simulink model "week2_problem4_2005052"  (R2021a)
settings: Solver=VariableStepAuto  StartTime=0.0  StopTime=10.0  RelTol=1e-3
model workspace (MAT data in the model file):
  B = 50
  J = Simulink.Parameter
  J.Value = 3.2284e-06
  J.DataType = 'auto'
  J.Dimensions = [1 1]
  Kd = 484.0516
  Ke = Simulink.Parameter
  Ke.Value = 0.0274
  Ke.DataType = 'auto'
  Ke.Dimensions = [1 1]
  Ki = 83.0917
  Kp = 495.0505
  Kt = Simulink.Parameter
  Kt.Value = 0.0274
  Kt.DataType = 'auto'
  Kt.Dimensions = [1 1]
  L = Simulink.Parameter
  L.Value = 2.75e-06
  L.DataType = 'auto'
  L.Dimensions = [1 1]
  M = 1000
  R = Simulink.Parameter
  R.Value = 4
  R.DataType = 'auto'
  R.Dimensions = [1 1]
  Ts = Simulink.Parameter
  Ts.Value = 0.01
  Ts.DataType = 'auto'
  Ts.Dimensions = [1 1]
  b = Simulink.Parameter
  b.Value = 3.5077e-06
  b.DataType = 'auto'
  b.Dimensions = [1 1]
  kd = Simulink.Parameter
  kd.Value = 50
  kd.DataType = 'auto'
  kd.Dimensions = [1 1]
  ki = Simulink.Parameter
  ki.Value = 22000
  ki.DataType = 'auto'
  ki.Dimensions = [1 1]
  kp = Simulink.Parameter
  kp.Value = 22000
  kp.DataType = 'auto'
  kp.Dimensions = [1 1]
settings Model: Creator=admin  LastModifiedBy=admin
settings SolverCC: AlgebraicLoopSolver=TrustRegion
settings DebuggingCC: SFMachineParentedDataDiag=warning

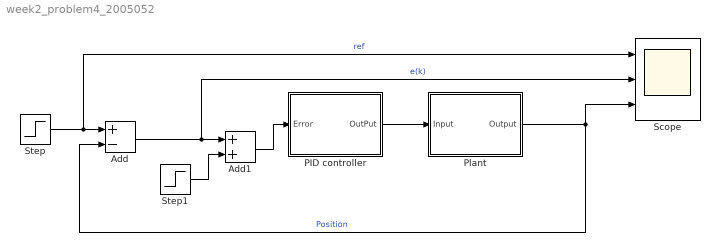
== system week2_problem4_2005052 ==
  Add : Sum  Inputs=+-
  Add1 : Sum
  PID controller : Subsystem  TreatAsAtomicUnit=on
  Plant : Subsystem
  Scope : Scope  NumInputPorts=3
  Step : Step  Time=0.01  SampleTime=0
  Step1 : Step  Time=0.01  After=0.1  SampleTime=0
  wires:
  Plant/1(Output) -> Add/2, Scope/3  "Position"
  Step/1 -> Scope/1, Add/1  "ref"
  Step1/1 -> Add1/2
  Add/1 -> Scope/2, Add1/1  "e(k)"
  Add1/1 -> PID controller/1(Error)
  PID controller/1(OutPut) -> Plant/1(Input)

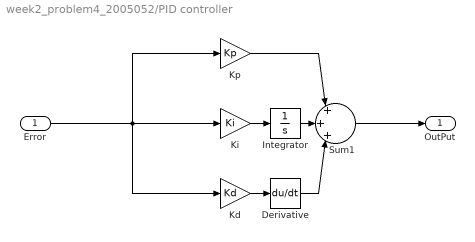
== system week2_problem4_2005052/PID controller ==
  Error : Inport  OutDataTypeStr=double  PortDimensions=1  SampleTime=0
  Derivative : Derivative
  Integrator : Integrator
  Kd : Gain  Gain=Kd
  Ki : Gain  Gain=Ki
  Kp : Gain  Gain=Kp
  Sum1 : Sum  Inputs=|+|+|+|
  OutPut : Outport  OutDataTypeStr=double  PortDimensions=1  SampleTime=0
  wires:
  Ki/1 -> Integrator/1
  Kd/1 -> Derivative/1
  Kp/1 -> Sum1/1
  Sum1/1 -> OutPut/1
  Error/1 -> Kd/1, Kp/1, Ki/1
  Derivative/1 -> Sum1/3
  Integrator/1 -> Sum1/2

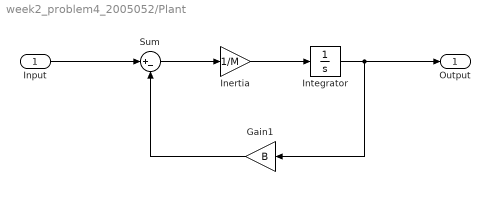
== system week2_problem4_2005052/Plant ==
  Input : Inport
  Gain1 : Gain  Gain=B
  Inertia : Gain  Gain=1/M
  Integrator : Integrator
  Sum : Sum  Inputs=|+-
  Output : Outport
  wires:
  Sum/1 -> Inertia/1
  Integrator/1 -> Output/1, Gain1/1
  Gain1/1 -> Sum/2
  Inertia/1 -> Integrator/1
  Input/1 -> Sum/1
